simulink model "StateDiagram2 copy"  (R2025b)
settings: Solver=FixedStepAuto  StartTime=0.0  StopTime=Inf  RelTol=1e-3
libraries: simulink_extras x1
settings Model: Creator=Soochan Kim  LastModifiedBy=Soochan Kim
settings OptimizationCC: OptimizeBlockIOStorage=off  OptimizeDataStoreBuffers=off  BusAssignmentInplaceUpdate=off
settings DebuggingCC: SFUnexpectedBacktrackingDiag=warning  SFNoUnconditionalDefaultTransitionDiag=warning
settings RTWCC: GenCodeOnly=on  GenerateReport=on  BuildConfiguration=Debug  LaunchReport=on
settings CodeAppCC: ForceParamTrailComments=on  MATLABSourceComments=on  EnableCustomComments=on
settings GRTTargetCC: MultiInstanceErrorCode=Warning  CombineSignalStateStructs=on  SupportVariableSizeSignals=on

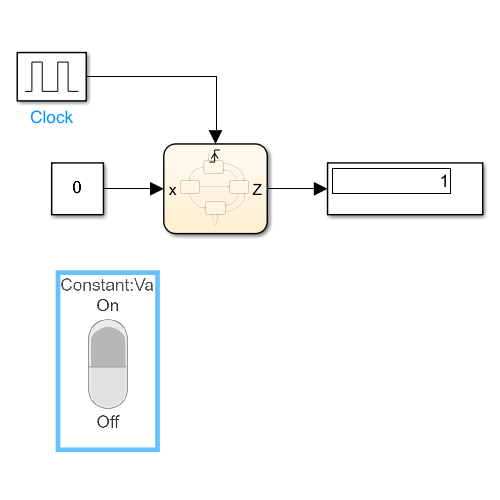
[thumbnail: Simulink's stored preview of the top-level diagram]
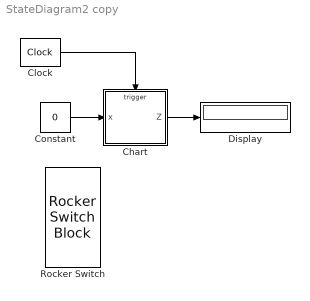
== system StateDiagram2 copy ==
  Chart : Stateflow chart  TreatAsAtomicUnit=on
  Clock : simulink_extras/Flip Flops/Clock  period=2
  Constant : Constant  Value=0
  Display : Display
  Rocker Switch : RockerSwitchBlock
  wires:
  Constant/1 -> Chart/1(x)
  Clock/1 -> Chart/Trigger
  Chart/1(Z) -> Display/1

== stateflow chart StateDiagram2 copy/Chart ==
  settings: executeAtInitialization=1
  state S0
    entry:
    Z=0
  state S3
    entry:
    Z=1
  state S1
    entry:
    Z=1
  state S2
    entry:
    Z=0
  (default) -> S0
  S0 -> S1 [order 2] : clk[x==1]
  S0 -> S3 [order 1] : clk[x==0]
  S1 -> S0 [order 1] : clk[x==0]
  S3 -> S1 [order 2] : clk[x==1]
  S3 -> S2 [order 1] : clk[x==0]
  S1 -> S2 [order 2] : clk[x==1]
  S2 -> S1 [order 1] : clk[x==0]
  S2 -> S2 [order 2] : clk[x==1]
  data: x input; Z output
  events: clk input RISING_EDGE_EVENT
